simulink model "modeloDiscreto_2022a"  (R2022a)
settings: Solver=FixedStepAuto  StartTime=0.0  StopTime=30  FixedStep=0.01  RelTol=1e-3
values from neighbouring files (symbols this model uses):
  A = [A11 A12; A21 A22]    [Identificacao.m]    (also in Linearizacao_CSTR.m; modeloDegrau.m = Ta*sum(y(1:tau+1)); parametrosFOPTD_igor.m = DeltaT*sum(y(1:k+1)))
  B = [B11 B12 B13 B14; B21 B22 B23 B24]    [Identificacao.m]    (also in Linearizacao_CSTR.m)
  C = [1 0]    [Identificacao.m]    (also in Linearizacao_CSTR.m)
  CA = 8.564    [Identificacao.m]    (also in Linearizacao_CSTR.m)
  D = [0 0 0 0]    [Identificacao.m]    (also in Linearizacao_CSTR.m)
  du1 = 0    [Identificacao.m]    (also in Linearizacao_CSTR.m = 0.01)
  du2 = 0    [Identificacao.m]    (also in Linearizacao_CSTR.m)
  du3 = 0    [Identificacao.m]    (also in Linearizacao_CSTR.m)
  du4 = 1    [Identificacao.m]    (also in Linearizacao_CSTR.m = 0)
  Gh1 = c2d(G, h1, 'zoh')    [Identificacao.m]    (also in Linearizacao_CSTR.m)
  Gh2 = c2d(G, h2, 'zoh')    [Identificacao.m]    (also in Linearizacao_CSTR.m)
  Gh3 = c2d(G, h3, 'zoh')    [Identificacao.m]    (also in Linearizacao_CSTR.m)
  h1 = 0.2    [Identificacao.m]    (also in Linearizacao_CSTR.m)
  h2 = 0.5    [Identificacao.m]    (also in Linearizacao_CSTR.m)
  h3 = 1.5    [Identificacao.m]    (also in Linearizacao_CSTR.m)
settings Model: Creator=egydi  LastModifiedBy=Mateus
settings SolverCC: AlgebraicLoopSolver=TrustRegion
settings DebuggingCC: UnconnectedInputMsg=warning  UnconnectedOutputMsg=warning  UnconnectedLineMsg=warning
settings RTWCC: DLArmComputeVersion=19.05

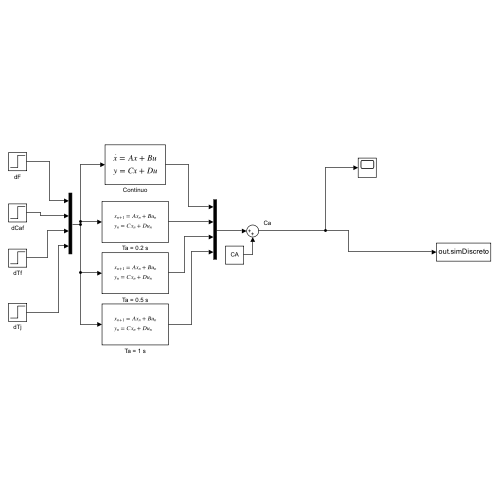
[thumbnail: Simulink's stored preview of the top-level diagram]
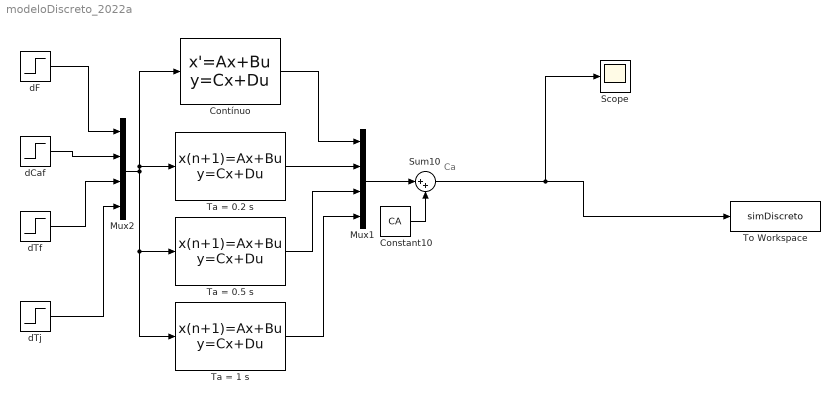
== system modeloDiscreto_2022a ==
  note: Ca
  Constant10 : Constant  Value=CA
  Contínuo : StateSpace  A=A  B=B  C=C  D=D  InitialCondition=0
  Mux1 : Mux
  Mux2 : Mux
  Scope : Scope
  Sum10 : Sum  Inputs=|++
  Ta = 0.2 s : DiscreteStateSpace  A=Gh1.A  B=Gh1.B  C=Gh1.C  D=Gh1.D  SampleTime=h1
  Ta = 0.5 s : DiscreteStateSpace  A=Gh2.A  B=Gh2.B  C=Gh2.C  D=Gh2.D  SampleTime=h2
  Ta = 1 s : DiscreteStateSpace  A=Gh3.A  B=Gh3.B  C=Gh3.C  D=Gh3.D  SampleTime=h3
  To Workspace : ToWorkspace  VariableName=simDiscreto  SaveFormat=Structure With Time  SampleTime=-1
  dCaf : Step  Time=0  After=du2  SampleTime=0
  dF : Step  Time=0  After=du1  SampleTime=0
  dTf : Step  Time=0  After=du3  SampleTime=0
  dTj : Step  Time=0  After=du4  SampleTime=0
  wires:
  Constant10/1 -> Sum10/2
  dCaf/1 -> Mux2/2
  dF/1 -> Mux2/1
  Mux2/1 -> Ta = 0.2 s/1, Contínuo/1, Ta = 0.5 s/1, Ta = 1 s/1
  Mux1/1 -> Sum10/1
  Contínuo/1 -> Mux1/1
  Ta = 0.5 s/1 -> Mux1/3
  Ta = 1 s/1 -> Mux1/4
  Ta = 0.2 s/1 -> Mux1/2
  Sum10/1 -> Scope/1, To Workspace/1
  dTf/1 -> Mux2/3
  dTj/1 -> Mux2/4
